simulink model "ComparatorTest"  (R2016a)
settings: Solver=VariableStepAuto  StartTime=0.0  StopTime=1  RelTol=1e-3
libraries: fl_lib x11, elec_lib x8, nesl_utility x4, powerlib_meascontrol x1
settings Model: Creator=Peter  LastModifiedBy=Peter

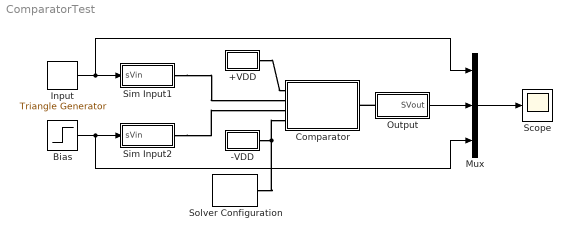
== system ComparatorTest ==
  +VDD : Subsystem
  -VDD : Subsystem
  Bias : Step  Time=0  After=.5  SampleTime=0
  Comparator : Subsystem
  Input : powerlib_meascontrol/Pulse & Signal Generators/Triangle Generator  Freq=2  Phase=0  Ts=0
  Mux : Mux  Inputs=3
  Output : Subsystem
  Scope : Scope
  Sim Input1 : Subsystem
  Sim Input2 : Subsystem
  Solver Configuration : nesl_utility/Solver Configuration  PhysicalDomain=network_engine_domain  SubClassName=solver  LeftPortType=input  RightPortType=generic  Accelerate=off  Tones=[]  Harmonics=[]  SimulateNoise=off  Profile=off  UseLocalSampling=off  EnableSwitchedLinearOptims=on  FrequencyDomain=off  UseCCode=off  RelTol=0.001  AbsTol=1e-06  MinStep=1e-09  ToWorkspace=off  RevertToSquareIcSolve=off  NumHomotopyIterations=100  PhasorMode=off  PhasorModeNumHarmonics=1  OverrideAbsTol=off  DoDC=off  ResidualTolerance=1e-09  UseLocalSolver=off  LocalSolverChoice=NE_BACKWARD_EULER_ADVANCER  LocalSolverSampleTime=0.001  DoFixedCost=off  MaxNonlinIter=3  MaxModeIter=2  LinearAlgebra=Sparse  DelaysMemoryBudget=1024  AutomaticFiltering=on  FilteringTimeConstant=0.001
  wires:
  Input/1 -> Mux/1, Sim Input1/1(sVin)
  Bias/1 -> Mux/3, Sim Input2/1(sVin)
  Mux/1 -> Scope/1
  Output/1(SVout) -> Mux/2
  connections:
  Solver Configuration/RConn1 -- -VDD/RConn1 -- Comparator/LConn4
  +VDD/RConn1 -- Comparator/LConn1
  Sim Input1/RConn1 -- Comparator/LConn2
  Output/LConn1 -- Comparator/RConn1
  Sim Input2/RConn1 -- Comparator/LConn3

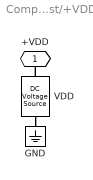
== system ComparatorTest/+VDD ==
  GND : fl_lib/Electrical/Electrical Elements/Electrical Reference
  VDD : fl_lib/Electrical/Electrical Sources/DC Voltage Source  v0=14.3 V
  +VDD : PMIOPort  Port=1  Side=Right
  connections:
  VDD/LConn1 -- +VDD/RConn1
  VDD/RConn1 -- GND/LConn1

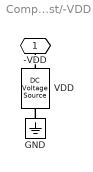
== system ComparatorTest/-VDD ==
  GND : fl_lib/Electrical/Electrical Elements/Electrical Reference
  VDD : fl_lib/Electrical/Electrical Sources/DC Voltage Source  v0=14.3 V
  -VDD : PMIOPort  Port=1  Side=Right
  connections:
  VDD/RConn1 -- -VDD/RConn1
  GND/LConn1 -- VDD/LConn1

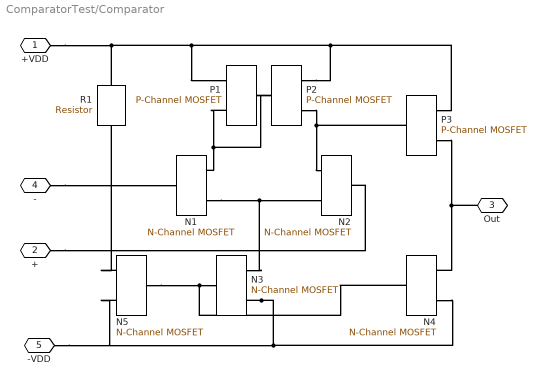
== system ComparatorTest/Comparator ==
  N{1..5} (5 alike) : elec_lib/Semiconductor Devices/N-Channel MOSFET  parameterization=1  prmDatasheet=1  prmEquCoeff=1  Beta=5 A/V^2  Rds=0.025 Ohm  Id=6 A  Vgs=10 V  Vth=1.7 V  lam=0 1/V  Tmeas=25 degC  RS=1e-4 Ohm  RD=0.01 Ohm  C_param=1  C_GS=270 pF  C_GD=80 pF  C_DS=0 pF  C_iss=350 pF  C_rss=80 pF  C_oss=0 pF  C_GS_vec=[ 270 300 290 280 295 255 ] pF  C_GD_vec=[ 450 400 300 190 95 55 ] pF  C_DS_vec=[ 450 410 390 230 175 115 ] pF  C_iss_vec=[ 720 700 590 470 390 310 ] pF  C_rss_vec=[ 450 400 300 190 95 55 ] pF  C_oss_vec=[ 900 810 690 420 270 170 ] pF  C_Vds_vec=[ 0.1 0.3 1 3 10 30 ] V  charge_linearity_param=1  C_OX=200 pF  V_C_OX=-0.5 V  dVth_dT=-6 mV/K  Rds_T2=0.037 Ohm  Tmeas2=125 degC  BEXDatasheet=-1.5  BEXEquCoeff=-1.5  TdeviceDatasheet=25 degC  TdeviceEquCoeff=25 degC  Rth=[ 0 10 ] K/W  thermal_mass_parameterization=1  thermal_mass=[ 0 1 ] J/K  thermal_time_constant=[ 0 10 ] s  thermal_mass_initial_temperatures=[ 25 25 ] degC
  P1 : elec_lib/Semiconductor Devices/P-Channel MOSFET  parameterization=1  prmDatasheet=1  prmEquCoeff=1  Beta=2 A/V^2  Rds=0.167 Ohm  Id=-2.5 A  Vgs=-4.5 V  Vth=-1.4 V  lam=0 1/V  Tmeas=25 degC  RS=1e-4 Ohm  RD=0.01 Ohm  C_param=1  C_GS=158 pF  C_GD=24 pF  C_DS=0 pF  C_iss=182 pF  C_rss=24 pF  C_oss=0 pF  C_GS_vec=[ 150 150 150 150 150 150 ] pF  C_GD_vec=[ 75 60 50 35 25 20 ] pF  C_DS_vec=[ 105 100 75 45 35 25 ] pF  C_iss_vec=[ 225 210 200 185 175 170 ] pF  C_rss_vec=[ 75 60 50 35 25 20 ] pF  C_oss_vec=[ 180 160 125 80 60 45 ] pF  C_Vsd_vec=[ 0.1 0.3 1 3 10 30 ] V  charge_linearity_param=1  C_OX=200 pF  V_C_OX=0.5 V  dVth_dT=2 mV/K  Rds_T2=0.25 Ohm  Tmeas2=125 degC  BEXDatasheet=-1.5  BEXEquCoeff=-1.5  TdeviceDatasheet=25 degC  TdeviceEquCoeff=25 degC  Rth=[ 0 10 ] K/W  thermal_mass_parameterization=1  thermal_mass=[ 0 1 ] J/K  thermal_time_constant=[ 0 10 ] s  thermal_mass_initial_temperatures=[ 25 25 ] degC
  P2 : elec_lib/Semiconductor Devices/P-Channel MOSFET  parameterization=1  prmDatasheet=1  prmEquCoeff=1  Beta=2 A/V^2  Rds=0.167 Ohm  Id=-2.5 A  Vgs=-4.5 V  Vth=-1.4 V  lam=0 1/V  Tmeas=25 degC  RS=1e-4 Ohm  RD=0.01 Ohm  C_param=1  C_GS=158 pF  C_GD=24 pF  C_DS=0 pF  C_iss=182 pF  C_rss=24 pF  C_oss=0 pF  C_GS_vec=[ 150 150 150 150 150 150 ] pF  C_GD_vec=[ 75 60 50 35 25 20 ] pF  C_DS_vec=[ 105 100 75 45 35 25 ] pF  C_iss_vec=[ 225 210 200 185 175 170 ] pF  C_rss_vec=[ 75 60 50 35 25 20 ] pF  C_oss_vec=[ 180 160 125 80 60 45 ] pF  C_Vsd_vec=[ 0.1 0.3 1 3 10 30 ] V  charge_linearity_param=1  C_OX=200 pF  V_C_OX=0.5 V  dVth_dT=2 mV/K  Rds_T2=0.25 Ohm  Tmeas2=125 degC  BEXDatasheet=-1.5  BEXEquCoeff=-1.5  TdeviceDatasheet=25 degC  TdeviceEquCoeff=25 degC  Rth=[ 0 10 ] K/W  thermal_mass_parameterization=1  thermal_mass=[ 0 1 ] J/K  thermal_time_constant=[ 0 10 ] s  thermal_mass_initial_temperatures=[ 25 25 ] degC
  P3 : elec_lib/Semiconductor Devices/P-Channel MOSFET  parameterization=1  prmDatasheet=1  prmEquCoeff=1  Beta=2 A/V^2  Rds=0.167 Ohm  Id=-2.5 A  Vgs=-4.5 V  Vth=-1.4 V  lam=0 1/V  Tmeas=25 degC  RS=1e-4 Ohm  RD=0.01 Ohm  C_param=1  C_GS=158 pF  C_GD=24 pF  C_DS=0 pF  C_iss=182 pF  C_rss=24 pF  C_oss=0 pF  C_GS_vec=[ 150 150 150 150 150 150 ] pF  C_GD_vec=[ 75 60 50 35 25 20 ] pF  C_DS_vec=[ 105 100 75 45 35 25 ] pF  C_iss_vec=[ 225 210 200 185 175 170 ] pF  C_rss_vec=[ 75 60 50 35 25 20 ] pF  C_oss_vec=[ 180 160 125 80 60 45 ] pF  C_Vsd_vec=[ 0.1 0.3 1 3 10 30 ] V  charge_linearity_param=1  C_OX=200 pF  V_C_OX=0.5 V  dVth_dT=2 mV/K  Rds_T2=0.25 Ohm  Tmeas2=125 degC  BEXDatasheet=-1.5  BEXEquCoeff=-1.5  TdeviceDatasheet=25 degC  TdeviceEquCoeff=25 degC  Rth=[ 0 10 ] K/W  thermal_mass_parameterization=1  thermal_mass=[ 0 1 ] J/K  thermal_time_constant=[ 0 10 ] s  thermal_mass_initial_temperatures=[ 25 25 ] degC
  R1 : fl_lib/Electrical/Electrical Elements/Resistor  R=70e3 Ohm  i_specify=off  i_priority=None  i=0 A  v_specify=off  v_priority=None  v=0 V
  +VDD : PMIOPort  Port=1  Side=Left
  + : PMIOPort  Port=2  Side=Left
  Out : PMIOPort  Port=3  Side=Right
  - : PMIOPort  Port=4  Side=Left
  -VDD : PMIOPort  Port=5  Side=Left
  connections:
  P1/RConn2 -- P2/LConn1 -- P1/LConn1 -- N1/RConn1
  P2/RConn2 -- P3/LConn1 -- N2/RConn1
  N5/RConn1 -- R1/RConn1
  N5/LConn1 -- N4/LConn1 -- N3/LConn1
  N3/RConn2 -- N4/RConn2 -- -VDD/RConn1 -- N5/RConn2
  P2/RConn1 -- P3/RConn1 -- P1/RConn1 -- R1/LConn1 -- +VDD/RConn1
  P3/RConn2 -- N4/RConn1 -- Out/RConn1
  N1/RConn2 -- N3/RConn1 -- N2/RConn2
  +/RConn1 -- N2/LConn1
  -/RConn1 -- N1/LConn1

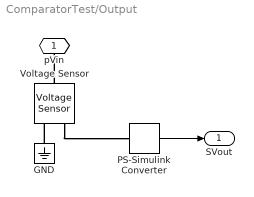
== system ComparatorTest/Output ==
  GND : fl_lib/Electrical/Electrical Elements/Electrical Reference
  PS-Simulink Converter : nesl_utility/PS-Simulink Converter  PhysicalDomain=network_engine_domain  SubClassName=ps_output  LeftPortType=input  RightPortType=output  PseudoPeriodic=off  Frequencies=[]  Unit=V  AffineConversion=off
  Voltage Sensor : fl_lib/Electrical/Electrical Sensors/Voltage Sensor
  pVin : PMIOPort  Port=1  Side=Left
  SVout : Outport
  wires:
  PS-Simulink Converter/1 -> SVout/1
  connections:
  GND/LConn1 -- Voltage Sensor/RConn2
  Voltage Sensor/LConn1 -- pVin/RConn1
  Voltage Sensor/RConn1 -- PS-Simulink Converter/LConn1

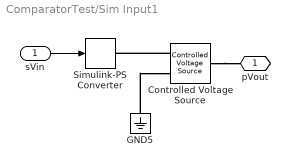
== system ComparatorTest/Sim Input1 ==
  sVin : Inport
  Controlled Voltage Source : fl_lib/Electrical/Electrical Sources/Controlled Voltage Source
  GND5 : fl_lib/Electrical/Electrical Elements/Electrical Reference
  Simulink-PS Converter : nesl_utility/Simulink-PS Converter  PhysicalDomain=network_engine_domain  SubClassName=ps_input  LeftPortType=input  RightPortType=output  PseudoPeriodic=off  Frequencies=[]  NoiseDistribution=none  NoiseParameters=[]  Unit=V  AffineConversion=off  InputFiltering=off  SimscapeFilterOrder=1  InputFilterTimeConstant=0.001  UdotUserProvided=1
  pVout : PMIOPort  Port=1  Side=Right
  wires:
  sVin/1 -> Simulink-PS Converter/1
  connections:
  Controlled Voltage Source/RConn1 -- Simulink-PS Converter/RConn1
  GND5/LConn1 -- Controlled Voltage Source/RConn2
  Controlled Voltage Source/LConn1 -- pVout/RConn1

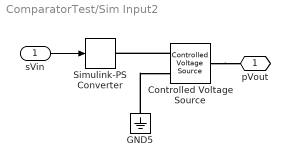
== system ComparatorTest/Sim Input2 ==
  sVin : Inport
  Controlled Voltage Source : fl_lib/Electrical/Electrical Sources/Controlled Voltage Source
  GND5 : fl_lib/Electrical/Electrical Elements/Electrical Reference
  Simulink-PS Converter : nesl_utility/Simulink-PS Converter  PhysicalDomain=network_engine_domain  SubClassName=ps_input  LeftPortType=input  RightPortType=output  PseudoPeriodic=off  Frequencies=[]  NoiseDistribution=none  NoiseParameters=[]  Unit=V  AffineConversion=off  InputFiltering=off  SimscapeFilterOrder=1  InputFilterTimeConstant=0.001  UdotUserProvided=1
  pVout : PMIOPort  Port=1  Side=Right
  wires:
  sVin/1 -> Simulink-PS Converter/1
  connections:
  Controlled Voltage Source/RConn1 -- Simulink-PS Converter/RConn1
  GND5/LConn1 -- Controlled Voltage Source/RConn2
  Controlled Voltage Source/LConn1 -- pVout/RConn1
